simulink model "hexacopter_sim"  (R2024b)
settings: Solver=VariableStepAuto  StartTime=0  StopTime=100  FixedStep=0.1  RelTol=1e-3  EnableMultiTasking=on
values from neighbouring files (symbols this model uses):
  A = [zeros(4), eye(4); zeros(4),zeros(4)]    [hexacopter_par.m]
  b = 1.177*10^-5    (= 1.177e-05)    [hexacopter_par.m]
  B = [zeros(4) ... (first row only)    [hexacopter_par.m]
  C_obs = eye(8)    [hexacopter_par.m]
  d = 1.855*10^-7    (= 1.855e-07)    [hexacopter_par.m]
  fault_level = 0    [hexacopter_par.m]
  g = 9.81    [hexacopter_par.m]
  Ic = Ic + temp    [hexacopter_par.m]
  Ix = Ic(1,1)    [hexacopter_par.m]
  Iy = Ic(2,2)    [hexacopter_par.m]
  Iz = Ic(3,3)    [hexacopter_par.m]
  J_T = 1/2 *m_r* R_r^2    (= 0.0001)    [hexacopter_par.m]
  K_lqr = lqr(A', C_obs', Q, R)'    [hexacopter_par.m]
  K_phi = 0.03    [hexacopter_par.m]
  K_psi = 0.1    [hexacopter_par.m]
  K_theta = 0.03    [hexacopter_par.m]
  Kx = .1    (= 0.1)    [hexacopter_par.m]
  Ky = .1    (= 0.1)    [hexacopter_par.m]
  Kz = .1    (= 0.1)    [hexacopter_par.m]
  L = 0.275    [hexacopter_par.m]
  m = 2.5    [hexacopter_par.m]
  M_RB = [ m*eye(3) , zeros(3) ; zeros(3) , Ic ]    [hexacopter_par.m]
  motor_index = 3    [hexacopter_par.m]
  T_psinv = pinv(T)    [hexacopter_par.m]
libraries: slpidlib x19, simulink_extras x17, aerolibutil x2, matrix_library x2, vrlib x2, slctrl_smc x1
(part 3 of 3)

== system hexacopter_sim/Flight Control System1/Outer loop position control ==
  Pos. refs : Inport
  eta : Inport  Port=2
  Demux : Demux
  Demux1 : Demux  Outputs=6
  Demux2 : Demux  Outputs=2
  Gain : Gain  Gain=-1
  MATLAB Function : MATLAB Function  TreatAsAtomicUnit=on
  Mux : Mux
  Mux1 : Mux  Inputs=2
  PID Controller : slpidlib/PID Controller  Controller=PID  Form=Parallel  TimeDomain=Continuous-time  UseExternalTs=off  SampleTime=-1  IntegratorMethod=Forward Euler  FilterMethod=Forward Euler  ControllerParametersSource=internal  P=10  I=0  UseKiTs=off  D=35  UseExternalDerivativeSource=off  N=110  UseFilter=on  TunerSelectOption=Transfer Function Based (PID Tuner App)  InitialConditionSource=internal  InitialConditionForIntegrator=0  InitialConditionForFilter=0  DifferentiatorICPrevScaledInput=0  ExternalReset=none  TrackingMode=off  Kt=1  LimitOutput=off  SatLimitsSource=internal  UpperSaturationLimit=100  LowerSaturationLimit=-100  LinearizeAsGain=on  AntiWindupMode=none  Kb=1  LimitIntegrator=off  UpperIntegratorSaturationLimit=inf  LowerIntegratorSaturationLimit=-inf  POutMin=[]  POutMax=[]  IOutMin=[]  IOutMax=[]  DOutMin=[]  DOutMax=[]  NOutMin=[]  NOutMax=[]  SumOutMin=[]  SumOutMax=[]  SaturationOutMin=[]  SaturationOutMax=[]  PParamMin=[]  PParamMax=[]  IParamMin=[]  IParamMax=[]  DParamMin=[]  DParamMax=[]  NParamMin=[]  NParamMax=[]  KbParamMin=[]  KbParamMax=[]  KtParamMin=[]  KtParamMax=[]  KbOutMin=[]  KbOutMax=[]  KtOutMin=[]  KtOutMax=[]  IntegratorOutMin=[]  IntegratorOutMax=[]  FilterOutMin=[]  FilterOutMax=[]  SumI1OutMin=[]  SumI1OutMax=[]  SumI2OutMin=[]  SumI2OutMax=[]  SumI3OutMin=[]  SumI3OutMax=[]  SumI4OutMin=[]  SumI4OutMax=[]  SumDOutMin=[]  SumDOutMax=[]  DifferentiatorOutMin=[]  DifferentiatorOutMax=[]  FilterDiffOutCoefMin=[]  FilterDiffOutCoefMax=[]  ReciprocalOutMin=[]  ReciprocalOutMax=[]  SumDenOutMin=[]  SumDenOutMax=[]  SumNumOutMin=[]  SumNumOutMax=[]  DivideOutMin=[]  DivideOutMax=[]  UdiffTsProdOutMin=[]  UdiffTsProdOutMax=[]  NTsProdOutMin=[]  NTsProdOutMax=[]  UintegralTsProdOutMin=[]  UintegralTsProdOutMax=[]  UngainTsProdOutMin=[]  UngainTsProdOutMax=[]  ClampingZeroOutDataTypeStr=Inherit: Inherit via back propagation  ClampingZeroOutMin=[]  ClampingZeroOutMax=[]  FilterDenConstantOutDataTypeStr=Inherit: Inherit via back propagation  FilterDenConstantOutMin=[]  FilterDenConstantOutMax=[]  PCopyOutDataTypeStr=Inherit: Inherit via back propagation  PCopyOutMin=[]  PCopyOutMax=[]  NCopyOutDataTypeStr=Inherit: Inherit via back propagation  NCopyOutMin=[]  NCopyOutMax=[]  IntegratorContinuousStateAttributes=''  IntegratorStateMustResolveToSignalObject=off  IntegratorRTWStateStorageClass=Auto  FilterContinuousStateAttributes=''  FilterStateMustResolveToSignalObject=off  FilterRTWStateStorageClass=Auto  ParallelPVariant=InternalParameters  IdealPVariant=Disabled  IVariant=InternalParameters  DVariant=InternalParameters  IntegratorVariant=Continuous  SatVariant=Disabled  AWVariant=Passthrough  PCopyVariant=Disabled  TRVariant=Disabled  FdbkBlocksVariant=Forward  IdealPFdbkVariant=Disabled  SatFdbkVariant=Disabled  DerivativeFilterVariant=ContFilter  NVariant=InternalParameters  NCopyVariant=Disabled  FilterICVariant=InternalICsFilter  IntegratorICVariant=InternalICs  ExternalResetVariant=Disabled  TRSumVariant=Passthrough  SumFdbkVariant=Disabled  SumVariant=Sum_PID  TsampFilterVariant=InternalTs  TsampNgainVariant=Passthrough  TsampIntegralVariant=Disabled_SignalSpec  ExternalSaturationOutDataTypeStr=Inherit: Same as second input  DerivativeSourceVariant=ErrorSignal  PreIntVariant=InternalPreInt
  PID Controller2 : slpidlib/PID Controller  Controller=PID  Form=Parallel  TimeDomain=Continuous-time  UseExternalTs=off  SampleTime=-1  IntegratorMethod=Forward Euler  FilterMethod=Forward Euler  ControllerParametersSource=internal  P=0.00012475905697814  I=1.47736767470013e-06  UseKiTs=off  D=0.00234086595699177  UseExternalDerivativeSource=off  N=231.972359946857  UseFilter=on  TunerSelectOption=Transfer Function Based (PID Tuner App)  InitialConditionSource=internal  InitialConditionForIntegrator=0  InitialConditionForFilter=0  DifferentiatorICPrevScaledInput=0  ExternalReset=none  TrackingMode=off  Kt=1  LimitOutput=off  SatLimitsSource=internal  UpperSaturationLimit=100  LowerSaturationLimit=-100  LinearizeAsGain=on  AntiWindupMode=none  Kb=1  LimitIntegrator=off  UpperIntegratorSaturationLimit=inf  LowerIntegratorSaturationLimit=-inf  POutMin=[]  POutMax=[]  IOutMin=[]  IOutMax=[]  DOutMin=[]  DOutMax=[]  NOutMin=[]  NOutMax=[]  SumOutMin=[]  SumOutMax=[]  SaturationOutMin=[]  SaturationOutMax=[]  PParamMin=[]  PParamMax=[]  IParamMin=[]  IParamMax=[]  DParamMin=[]  DParamMax=[]  NParamMin=[]  NParamMax=[]  KbParamMin=[]  KbParamMax=[]  KtParamMin=[]  KtParamMax=[]  KbOutMin=[]  KbOutMax=[]  KtOutMin=[]  KtOutMax=[]  IntegratorOutMin=[]  IntegratorOutMax=[]  FilterOutMin=[]  FilterOutMax=[]  SumI1OutMin=[]  SumI1OutMax=[]  SumI2OutMin=[]  SumI2OutMax=[]  SumI3OutMin=[]  SumI3OutMax=[]  SumI4OutMin=[]  SumI4OutMax=[]  SumDOutMin=[]  SumDOutMax=[]  DifferentiatorOutMin=[]  DifferentiatorOutMax=[]  FilterDiffOutCoefMin=[]  FilterDiffOutCoefMax=[]  ReciprocalOutMin=[]  ReciprocalOutMax=[]  SumDenOutMin=[]  SumDenOutMax=[]  SumNumOutMin=[]  SumNumOutMax=[]  DivideOutMin=[]  DivideOutMax=[]  UdiffTsProdOutMin=[]  UdiffTsProdOutMax=[]  NTsProdOutMin=[]  NTsProdOutMax=[]  UintegralTsProdOutMin=[]  UintegralTsProdOutMax=[]  UngainTsProdOutMin=[]  UngainTsProdOutMax=[]  ClampingZeroOutDataTypeStr=Inherit: Inherit via back propagation  ClampingZeroOutMin=[]  ClampingZeroOutMax=[]  FilterDenConstantOutDataTypeStr=Inherit: Inherit via back propagation  FilterDenConstantOutMin=[]  FilterDenConstantOutMax=[]  PCopyOutDataTypeStr=Inherit: Inherit via back propagation  PCopyOutMin=[]  PCopyOutMax=[]  NCopyOutDataTypeStr=Inherit: Inherit via back propagation  NCopyOutMin=[]  NCopyOutMax=[]  IntegratorContinuousStateAttributes=''  IntegratorStateMustResolveToSignalObject=off  IntegratorRTWStateStorageClass=Auto  FilterContinuousStateAttributes=''  FilterStateMustResolveToSignalObject=off  FilterRTWStateStorageClass=Auto  ParallelPVariant=InternalParameters  IdealPVariant=Disabled  IVariant=InternalParameters  DVariant=InternalParameters  IntegratorVariant=Continuous  SatVariant=Disabled  AWVariant=Passthrough  PCopyVariant=Disabled  TRVariant=Disabled  FdbkBlocksVariant=Forward  IdealPFdbkVariant=Disabled  SatFdbkVariant=Disabled  DerivativeFilterVariant=ContFilter  NVariant=InternalParameters  NCopyVariant=Disabled  FilterICVariant=InternalICsFilter  IntegratorICVariant=InternalICs  ExternalResetVariant=Disabled  TRSumVariant=Passthrough  SumFdbkVariant=Disabled  SumVariant=Sum_PID  TsampFilterVariant=InternalTs  TsampNgainVariant=Passthrough  TsampIntegralVariant=Disabled_SignalSpec  ExternalSaturationOutDataTypeStr=Inherit: Same as second input  DerivativeSourceVariant=ErrorSignal  PreIntVariant=InternalPreInt
  Sum : Sum  Inputs=|+-
  Sum1 : Sum  Inputs=|+-
  Terminator : Terminator
  Terminator1 : Terminator
  Terminator2 : Terminator
  desired z,phi,theta,psi : Outport
  wires:
  Demux1/6 -> MATLAB Function/2(psi)
  Demux1/5 -> Terminator2/1
  Demux2/2 -> PID Controller2/1
  Demux2/1 -> PID Controller/1
  Mux1/1 -> MATLAB Function/1(Deltap_e)
  MATLAB Function/1(Deltap_b) -> Demux2/1
  Sum1/1 -> Mux1/2
  Sum/1 -> Mux1/1
  Demux/2 -> Sum1/1
  Demux/1 -> Sum/1
  Demux/4 -> Mux/4
  Demux/3 -> Mux/1
  PID Controller2/1 -> Mux/2
  Gain/1 -> Mux/3
  PID Controller/1 -> Gain/1
  Mux/1 -> desired z,phi,theta,psi/1
  eta/1 -> Demux1/1
  Demux1/1 -> Sum/2
  Demux1/4 -> Terminator1/1
  Demux1/2 -> Sum1/2
  Pos. refs/1 -> Demux/1
  Demux1/3 -> Terminator/1

== system hexacopter_sim/Formatting/Axes to VR Axes ==
  Xe : Inport
  Demux : Demux  Outputs=3
      settings: DisplayOption=none
  Mux : Mux  Inputs=3
  rad-->deg1 : Gain  SaturateOnIntegerOverflow=on  OutDataTypeStr=Inherit: Same as input  ParamDataTypeStr=Inherit: Same as input
  Xe VR : Outport  VectorParamsAs1DForOutWhenUnconnected=off
  wires:
  Xe/1 -> Demux/1
  Demux/1 -> Mux/1
  Demux/3 -> rad-->deg1/1
  Mux/1 -> Xe VR/1
  Demux/2 -> Mux/2
  rad-->deg1/1 -> Mux/3

== system hexacopter_sim/Formatting/Euler to VR ==
  Euler Angles : Inport
  Axis Angle Vector : Subsystem
  Mux : Mux  Inputs=2
  Mux1 : Mux  Inputs=2
  Mux2 : Mux  Inputs=2
  Quaternion Multiplication (Pitch & Yaw) : aerolibutil/Quaternion Multiplication
  Quaternion Multiplication (Roll) : aerolibutil/Quaternion Multiplication
  Quaternion Normalization : Subsystem
  Quaternion Normalization1 : Subsystem
  Quaternion Normalization2 : Subsystem
  Selector : Selector  InputPortWidth=3  IndexOptions=Index vector (dialog)  Indices=[3]  OutputSizes=1
  Selector1 : Selector  InputPortWidth=3  IndexOptions=Index vector (dialog)  Indices=[2]  OutputSizes=1
  Selector2 : Selector  InputPortWidth=3  IndexOptions=Index vector (dialog)  Indices=[1]  OutputSizes=1
  Vr Pitch Axes : Constant  Value=[0 0 1]
  Vr Roll Axes : Constant  Value=[1 0 0]
  Vr Yaw Axes : Constant  Value=[0 -1 0]
  Axis Angle : Outport  VectorParamsAs1DForOutWhenUnconnected=off
  wires:
  Quaternion Multiplication (Roll)/1 -> Axis Angle Vector/1(e0)
  Axis Angle Vector/1(e0_norm) -> Axis Angle/1
  Quaternion Normalization/1(e0_norm) -> Quaternion Multiplication (Roll)/2
  Quaternion Normalization2/1(e0_norm) -> Quaternion Multiplication (Pitch & Yaw)/1
  Quaternion Normalization1/1(e0_norm) -> Quaternion Multiplication (Pitch & Yaw)/2
  Mux2/1 -> Quaternion Normalization2/1(e0)
  Mux1/1 -> Quaternion Normalization1/1(e0)
  Mux/1 -> Quaternion Normalization/1(e0)
  Selector/1 -> Mux2/1
  Vr Yaw Axes/1 -> Mux2/2
  Selector1/1 -> Mux1/1
  Vr Pitch Axes/1 -> Mux1/2
  Selector2/1 -> Mux/1
  Vr Roll Axes/1 -> Mux/2
  Euler Angles/1 -> Selector2/1, Selector1/1, Selector/1
  Quaternion Multiplication (Pitch & Yaw)/1 -> Quaternion Multiplication (Roll)/1

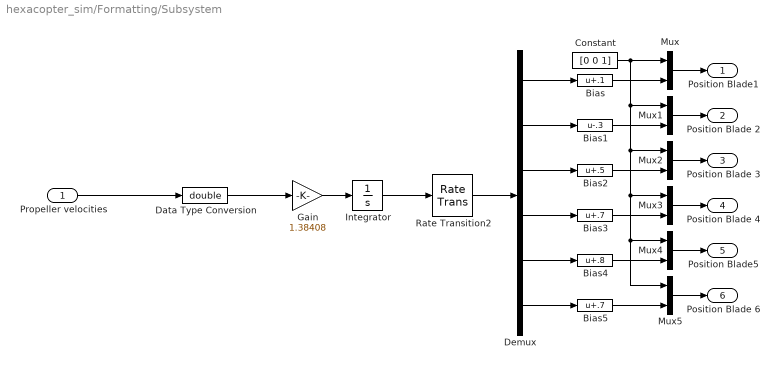
== system hexacopter_sim/Formatting/Subsystem ==
  Propeller velocities : Inport
  Bias : Bias  Bias=.1  SaturateOnIntegerOverflow=off
  Bias1 : Bias  Bias=-.3  SaturateOnIntegerOverflow=off
  Bias2 : Bias  Bias=.5  SaturateOnIntegerOverflow=off
  Bias3 : Bias  Bias=.7  SaturateOnIntegerOverflow=off
  Bias4 : Bias  Bias=.8  SaturateOnIntegerOverflow=off
  Bias5 : Bias  Bias=.7  SaturateOnIntegerOverflow=off
  Constant : Constant  Value=[0 0 1]
  Data Type Conversion : DataTypeConversion  OutDataTypeStr=double  SaturateOnIntegerOverflow=off  RndMeth=Floor
  Demux : Demux  Outputs=6
  Gain : Gain  Gain=1.38408
  Integrator : Integrator  InitialCondition=[.1 ; .2 ;-.3 ;-.4;.5;.6]  WrapState=on  WrappedStateUpperValue=2*pi  WrappedStateLowerValue=-2*pi
  Mux{,1..5} (6 alike) : Mux  Inputs=2
  Rate Transition2 : RateTransition
  Position Blade1 : Outport  VectorParamsAs1DForOutWhenUnconnected=off
  Position Blade 2 : Outport  Port=2  VectorParamsAs1DForOutWhenUnconnected=off
  Position Blade 3 : Outport  Port=3  VectorParamsAs1DForOutWhenUnconnected=off
  Position Blade 4 : Outport  Port=4  VectorParamsAs1DForOutWhenUnconnected=off
  Position Blade5 : Outport  Port=5  VectorParamsAs1DForOutWhenUnconnected=off
  Position Blade 6 : Outport  Port=6  VectorParamsAs1DForOutWhenUnconnected=off
  wires:
  Bias3/1 -> Mux3/2
  Mux3/1 -> Position Blade 4/1
  Bias1/1 -> Mux1/2
  Bias2/1 -> Mux2/2
  Demux/2 -> Bias1/1
  Constant/1 -> Mux4/1, Mux5/1, Mux3/1, Mux2/1, Mux1/1, Mux/1
  Mux1/1 -> Position Blade 2/1
  Mux2/1 -> Position Blade 3/1
  Integrator/1 -> Rate Transition2/1
  Mux/1 -> Position Blade1/1
  Demux/3 -> Bias2/1
  Bias/1 -> Mux/2
  Propeller velocities/1 -> Data Type Conversion/1
  Demux/4 -> Bias3/1
  Rate Transition2/1 -> Demux/1
  Demux/1 -> Bias/1
  Data Type Conversion/1 -> Gain/1
  Gain/1 -> Integrator/1
  Mux4/1 -> Position Blade5/1
  Mux5/1 -> Position Blade 6/1
  Demux/5 -> Bias4/1
  Demux/6 -> Bias5/1
  Bias5/1 -> Mux5/2
  Bias4/1 -> Mux4/2

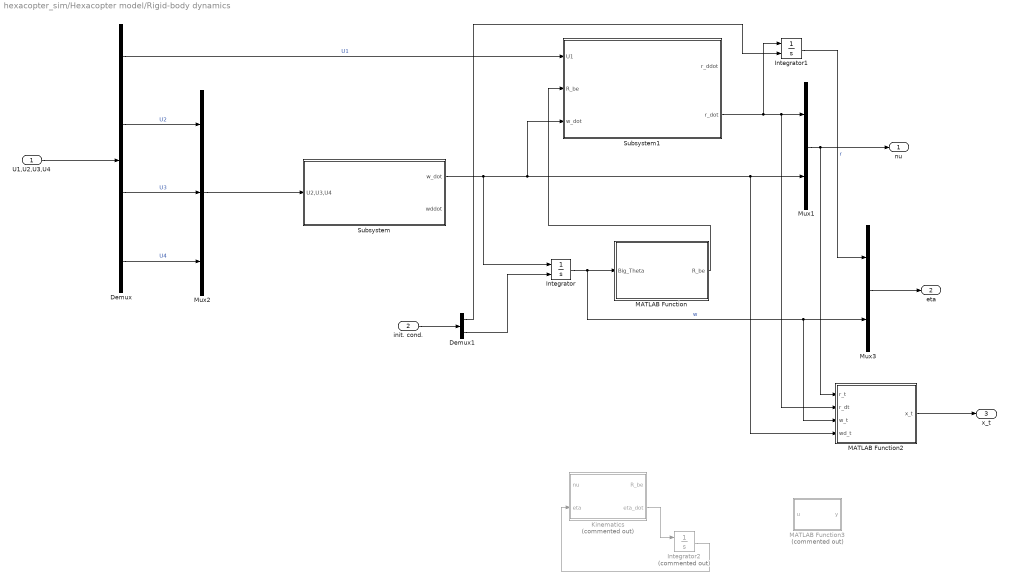
== system hexacopter_sim/Hexacopter model/Rigid-body dynamics ==
  U1,U2,U3,U4 : Inport
  init. cond. : Inport  Port=2
  Demux : Demux
  Demux1 : Demux  Outputs=2
  Integrator : Integrator  InitialConditionSource=external
  Integrator1 : Integrator  InitialConditionSource=external
  Integrator2 : Integrator  Commented=on  InitialConditionSource=external  InitialCondition=[0;0;-10;0;pi/2;0]
  Kinematics : MATLAB Function  Commented=on  TreatAsAtomicUnit=on
  MATLAB Function : MATLAB Function  TreatAsAtomicUnit=on
  MATLAB Function2 : MATLAB Function  TreatAsAtomicUnit=on
  MATLAB Function3 : MATLAB Function  Commented=on  TreatAsAtomicUnit=on
  Mux1 : Mux  Inputs=2
  Mux2 : Mux  Inputs=3
  Mux3 : Mux  Inputs=2
  Subsystem : Subsystem
  Subsystem1 : Subsystem
  nu : Outport
  eta : Outport  Port=2
  x_t : Outport  Port=3
  wires:
  U1,U2,U3,U4/1 -> Demux/1
  Demux/2 -> Mux2/1  "U2"
  Demux/3 -> Mux2/2  "U3"
  Demux/4 -> Mux2/3  "U4"
  Mux1/1 -> MATLAB Function2/1(r_t), nu/1
  Mux2/1 -> Subsystem/1(U2,U3,U4)
  Demux/1 -> Subsystem1/1(U1)  "U1"
  Subsystem/1(w_dot) -> Integrator/1, Subsystem1/3(w_dot), MATLAB Function2/4(wd_t), Mux1/2
  Subsystem1/2(r_dot) -> Integrator1/1, MATLAB Function2/2(r_dt), Mux1/1
  Integrator/1 -> MATLAB Function2/3(w_t), Mux3/2, MATLAB Function/1(Big_Theta)  "w"
  MATLAB Function/1(R_be) -> Subsystem1/2(R_be)
  Integrator1/1 -> Mux3/1  "r"
  Mux3/1 -> eta/1
  init. cond./1 -> Demux1/1
  Demux1/2 -> Integrator/2
  Demux1/1 -> Integrator1/2
  MATLAB Function2/1(x_t) -> x_t/1
  Integrator2/1 -> Kinematics/2(eta)
  Kinematics/2(eta_dot) -> Integrator2/1

== system hexacopter_sim/Observer - Allocation Matrix/U1 ==
  Fi : Inport
  Demux : Demux  Outputs=6
  Sum of Elements : Sum  Inputs=++++++
  U1 : Outport
  wires:
  Fi/1 -> Demux/1
  Demux/2 -> Sum of Elements/2  "F2"
  Demux/1 -> Sum of Elements/1  "F1"
  Demux/3 -> Sum of Elements/3  "F3"
  Demux/4 -> Sum of Elements/4  "F4"
  Demux/5 -> Sum of Elements/5  "F5"
  Demux/6 -> Sum of Elements/6  "F6"
  Sum of Elements/1 -> U1/1

== system hexacopter_sim/Observer - Allocation Matrix/U2 ==
  Fi : Inport
  Demux : Demux  Outputs=6
  Gain : Gain  Gain=1/2
  Gain1 : Gain  Gain=L
  Sum : Sum  Inputs=|-+
  Sum of Elements : Sum  Inputs=-++-
  Sum1 : Sum  Inputs=|++
  U2 : Outport
  wires:
  Fi/1 -> Demux/1
  Demux/1 -> Sum/1  "F1"
  Demux/6 -> Sum of Elements/4  "F6"
  Demux/5 -> Sum of Elements/3  "F5"
  Sum of Elements/1 -> Gain/1
  Sum/1 -> Sum1/1
  Gain/1 -> Sum1/2
  Sum1/1 -> Gain1/1
  Gain1/1 -> U2/1
  Demux/2 -> Sum of Elements/1  "F2"
  Demux/4 -> Sum/2  "F4"
  Demux/3 -> Sum of Elements/2  "F3"

== system hexacopter_sim/Observer - Allocation Matrix/U3 ==
  Fi : Inport
  Demux : Demux  Outputs=6
  Gain : Gain  Gain=L/2*sqrt(3)
  Sum of Elements : Sum  Inputs=++--
  Terminator : Terminator
  Terminator1 : Terminator
  U3 : Outport
  wires:
  Sum of Elements/1 -> Gain/1
  Demux/5 -> Sum of Elements/3  "F5"
  Demux/6 -> Sum of Elements/4  "F6"
  Fi/1 -> Demux/1
  Demux/1 -> Terminator/1  "F1"
  Demux/2 -> Sum of Elements/1  "F2"
  Gain/1 -> U3/1
  Demux/4 -> Terminator1/1  "F4"
  Demux/3 -> Sum of Elements/2  "F3"

== system hexacopter_sim/Observer - Allocation Matrix/U4 ==
  Tau_i : Inport
  Demux : Demux  Outputs=6
  Sum of Elements : Sum  Inputs=-+--++
  U4 : Outport
  wires:
  Tau_i/1 -> Demux/1
  Sum of Elements/1 -> U4/1
  Demux/1 -> Sum of Elements/1  "Tau_1"
  Demux/2 -> Sum of Elements/2  "Tau_2"
  Demux/3 -> Sum of Elements/3  "Tau_3"
  Demux/4 -> Sum of Elements/4  "Tau_4"
  Demux/5 -> Sum of Elements/5  "Tau_5"
  Demux/6 -> Sum of Elements/6  "Tau_6"

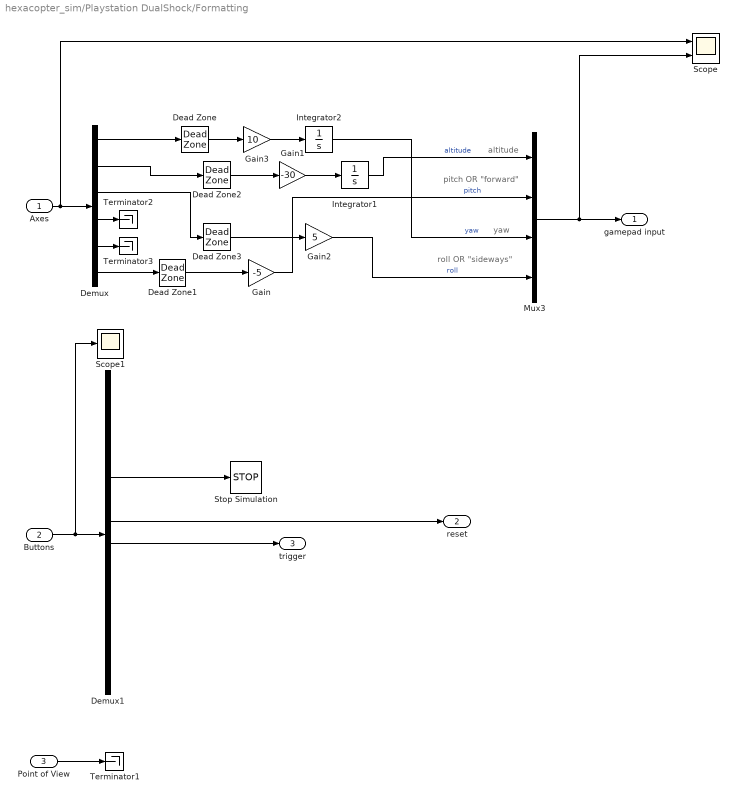
== system hexacopter_sim/Playstation DualShock/Formatting ==
  note: roll OR "sideways"
  note: altitude
  note: pitch OR "forward"
  note: yaw
  Axes : Inport
  Buttons : Inport  Port=2
  Point of View : Inport  Port=3
  Dead Zone{,1..3} (4 alike) : DeadZone  LowerValue=-0.2  UpperValue=0.2
  Demux : Demux  Outputs=6
  Demux1 : Demux  Outputs=14
  Gain : Gain  Gain=-5
  Gain1 : Gain  Gain=-30
  Gain2 : Gain  Gain=5
  Gain3 : Gain  Gain=10
  Integrator1 : Integrator  InitialCondition=10
  Integrator2 : Integrator
  Mux3 : Mux
  Scope : Scope  NumInputPorts=2
  Scope1 : Scope
  Stop Simulation : Stop
  Terminator1 : Terminator
  Terminator2 : Terminator
  Terminator3 : Terminator
  gamepad input : Outport
  reset : Outport  Port=2
  trigger : Outport  Port=3
  wires:
  Mux3/1 -> Scope/2, gamepad input/1
  Axes/1 -> Scope/1, Demux/1
  Demux/1 -> Dead Zone/1
  Dead Zone1/1 -> Gain/1
  Demux/2 -> Dead Zone2/1
  Dead Zone2/1 -> Gain1/1
  Dead Zone/1 -> Gain3/1
  Dead Zone3/1 -> Gain2/1
  Point of View/1 -> Terminator1/1
  Gain1/1 -> Integrator1/1
  Gain3/1 -> Integrator2/1
  Demux/3 -> Dead Zone3/1
  Integrator1/1 -> Mux3/1  "altitude"
  Gain2/1 -> Mux3/4  "roll"
  Gain/1 -> Mux3/2  "pitch"
  Integrator2/1 -> Mux3/3  "yaw"
  Demux/6 -> Dead Zone1/1
  Demux/4 -> Terminator2/1
  Demux/5 -> Terminator3/1
  Buttons/1 -> Scope1/1, Demux1/1
  Demux1/8 -> trigger/1
  Demux1/7 -> reset/1
  Demux1/5 -> Stop Simulation/1

== system hexacopter_sim/Quadcopter model/Kinematics ==
  nu : Inport
  init. cond. : Inport  Port=2
  Integrator : Integrator  InitialConditionSource=external  InitialCondition=[0;0;-10;0;pi/2;0]
  Kinematics : MATLAB Function  TreatAsAtomicUnit=on
  R_be : Outport
  eta : Outport  Port=2
  wires:
  Kinematics/1(R_be) -> R_be/1
  Kinematics/2(eta_dot) -> Integrator/1
  nu/1 -> Kinematics/1(nu)
  init. cond./1 -> Integrator/2
  Integrator/1 -> eta/1, Kinematics/2(eta)

== system hexacopter_sim/Quadcopter model/Rigid-body dynamics ==
  note: $\nu$
  tau_g : Inport
  tau_p : Inport  Port=2
  Constant : Constant  Value=m
  Constant1 : Constant  Value=Ic  VectorParams1D=off
  Coriolis term : MATLAB Function  TreatAsAtomicUnit=on
  Gain : Gain  Gain=inv(M_RB)  Multiplication=Matrix(K*u) (u vector)
  Integrator1 : Integrator  InitialCondition=[0;0;0;0;0;0]
  Sum : Sum  Inputs=++-
  nu : Outport
  wires:
  Integrator1/1 -> nu/1, Coriolis term/1(nu)
  Constant/1 -> Coriolis term/2(m)
  Sum/1 -> Gain/1
  tau_p/1 -> Sum/2
  Coriolis term/1(Cnunu) -> Sum/3
  Constant1/1 -> Coriolis term/3(Ic)
  Gain/1 -> Integrator1/1
  tau_g/1 -> Sum/1

== system hexacopter_sim/Quadcopter model/gravity ==
  R_be : Inport
  Manual Switch : ManualSwitch
  Math Function : Math  Operator=transpose
  Matrix Multiply : Product  Multiplication=Matrix(*)
  Mux2 : Mux  Inputs=2
  gravity vector : Constant  Value=[0;0;-m*g]  VectorParams1D=off
  zeros : Constant  Value=[0;0;0]  VectorParams1D=off
  tau_g : Outport
  wires:
  Matrix Multiply/1 -> Manual Switch/1
  Manual Switch/1 -> Mux2/1
  Mux2/1 -> tau_g/1
  gravity vector/1 -> Matrix Multiply/2
  zeros/1 -> Mux2/2, Manual Switch/2
  Math Function/1 -> Matrix Multiply/1
  R_be/1 -> Math Function/1

== system hexacopter_sim/Formatting/Euler to VR/Axis Angle Vector ==
  e0 : Inport
  2 : Gain  Gain=2  SaturateOnIntegerOverflow=on  OutDataTypeStr=Inherit: Same as input  ParamDataTypeStr=Inherit: Same as input
  Constant : Constant  Value=1e-6
  Demux : Demux  Outputs=[1 3 ]
      settings: DisplayOption=none
  Mux : Mux  Inputs=2
  Product : Product  Inputs=*/  InputSameDT=on  SaturateOnIntegerOverflow=on  OutDataTypeStr=Inherit: Same as first input
  Switch : Switch  Criteria=u2 ~= 0  SaturateOnIntegerOverflow=off  InputSameDT=off
  Trigonometric Function : Trigonometry
  Trigonometric Function2 : Trigonometry  Operator=acos
  e0_norm : Outport  VectorParamsAs1DForOutWhenUnconnected=off
  wires:
  Demux/1 -> Trigonometric Function2/1
  Demux/2 -> Product/1
  Mux/1 -> e0_norm/1
  Product/1 -> Mux/1
  2/1 -> Mux/2
  Trigonometric Function/1 -> Switch/1, Switch/2
  Trigonometric Function2/1 -> Trigonometric Function/1, 2/1
  e0/1 -> Demux/1
  Constant/1 -> Switch/3
  Switch/1 -> Product/2

== system hexacopter_sim/Formatting/Euler to VR/Quaternion Normalization ==
  e0 : Inport
  1/2 : Gain  Gain=1/2  SaturateOnIntegerOverflow=on  OutDataTypeStr=Inherit: Same as input  ParamDataTypeStr=Inherit: Same as input
  Demux : Demux  Outputs=[1 3]
      settings: DisplayOption=none
  Mux : Mux  Inputs=2
  Product : Product  InputSameDT=on  SaturateOnIntegerOverflow=on  OutDataTypeStr=Inherit: Same as first input
  Trigonometric Function : Trigonometry
  Trigonometric Function1 : Trigonometry  Operator=cos
  e0_norm : Outport  VectorParamsAs1DForOutWhenUnconnected=off
  wires:
  Trigonometric Function1/1 -> Mux/1
  Demux/2 -> Product/2
  Demux/1 -> 1/2/1
  Mux/1 -> e0_norm/1
  Product/1 -> Mux/2
  Trigonometric Function/1 -> Product/1
  1/2/1 -> Trigonometric Function1/1, Trigonometric Function/1
  e0/1 -> Demux/1

== system hexacopter_sim/Formatting/Euler to VR/Quaternion Normalization1 ==
  e0 : Inport
  1/2 : Gain  Gain=1/2  SaturateOnIntegerOverflow=on  OutDataTypeStr=Inherit: Same as input  ParamDataTypeStr=Inherit: Same as input
  Demux : Demux  Outputs=[1 3]
      settings: DisplayOption=none
  Mux : Mux  Inputs=2
  Product : Product  InputSameDT=on  SaturateOnIntegerOverflow=on  OutDataTypeStr=Inherit: Same as first input
  Trigonometric Function : Trigonometry
  Trigonometric Function1 : Trigonometry  Operator=cos
  e0_norm : Outport  VectorParamsAs1DForOutWhenUnconnected=off
  wires:
  e0/1 -> Demux/1
  1/2/1 -> Trigonometric Function/1, Trigonometric Function1/1
  Trigonometric Function/1 -> Product/1
  Product/1 -> Mux/2
  Mux/1 -> e0_norm/1
  Demux/1 -> 1/2/1
  Demux/2 -> Product/2
  Trigonometric Function1/1 -> Mux/1

== system hexacopter_sim/Formatting/Euler to VR/Quaternion Normalization2 ==
  e0 : Inport
  1/2 : Gain  Gain=1/2  SaturateOnIntegerOverflow=on  OutDataTypeStr=Inherit: Same as input  ParamDataTypeStr=Inherit: Same as input
  Demux : Demux  Outputs=[1 3]
      settings: DisplayOption=none
  Mux : Mux  Inputs=2
  Product : Product  InputSameDT=on  SaturateOnIntegerOverflow=on  OutDataTypeStr=Inherit: Same as first input
  Trigonometric Function : Trigonometry
  Trigonometric Function1 : Trigonometry  Operator=cos
  e0_norm : Outport  VectorParamsAs1DForOutWhenUnconnected=off
  wires:
  Trigonometric Function1/1 -> Mux/1
  Demux/2 -> Product/2
  Demux/1 -> 1/2/1
  Mux/1 -> e0_norm/1
  Product/1 -> Mux/2
  Trigonometric Function/1 -> Product/1
  1/2/1 -> Trigonometric Function1/1, Trigonometric Function/1
  e0/1 -> Demux/1

== system hexacopter_sim/Hexacopter model/Rigid-body dynamics/Subsystem ==
  U2,U3,U4 : Inport
  Constant : Constant  Value=Ic
  Cross Product : matrix_library/Cross Product
  Integrator : Integrator  InitialCondition=[0;0;0]
  Matrix Multiply1 : Product  Multiplication=Matrix(*)
  Sum : Sum  Inputs=|+-
  w_dot : Outport
  wddot : Outport  Port=2
  wires:
  Sum/1 -> Matrix Multiply1/2, wddot/1, Integrator/1  "wddot"
  Cross Product/1 -> Sum/2
  Integrator/1 -> Cross Product/1, w_dot/1  "w_dot"
  U2,U3,U4/1 -> Sum/1
  Matrix Multiply1/1 -> Cross Product/2
  Constant/1 -> Matrix Multiply1/1

== system hexacopter_sim/Hexacopter model/Rigid-body dynamics/Subsystem1 ==
  U1 : Inport
  R_be : Inport  Port=2
  w_dot : Inport  Port=3
  Constant2 : Constant  Value=[0;0]  VectorParams1D=off
  Cross Product1 : matrix_library/Cross Product
  Gain : Gain  Gain=1/m
  Integrator : Integrator  InitialCondition=[0;0;0]
  Matrix Multiply : Product  Multiplication=Matrix(*)
  Mux : Mux  Inputs=2
  Sum of Elements : Sum  Inputs=+--
  gravity vector : Constant  Value=[0;0;m*g]  VectorParams1D=off
  r_ddot : Outport
  r_dot : Outport  Port=2
  wires:
  Sum of Elements/1 -> Cross Product1/1, Gain/1
  gravity vector/1 -> Sum of Elements/2
  Constant2/1 -> Mux/1
  Gain/1 -> Integrator/1, r_ddot/1  "r_ddot"
  Matrix Multiply/1 -> Sum of Elements/1
  Cross Product1/1 -> Sum of Elements/3
  U1/1 -> Mux/2
  w_dot/1 -> Cross Product1/2
  Integrator/1 -> r_dot/1
  Mux/1 -> Matrix Multiply/2
  R_be/1 -> Matrix Multiply/1  "R_be"

== matlab function hexacopter_sim/Hexacopter model/Rigid-body dynamics/MATLAB Function2 ==
  data: r_t input; r_dt input; w_t input; wd_t input; x_t output
function x_t = fcn(r_t,r_dt,w_t,wd_t)

% Extract position components
% x = r_t(1); % x-coordinate
% y = r_t(2); % y-coordinate
z = r_t(3); % z-coordinate

% Extract velocity components
% dx = r_dt(1); % x-velocity
% dy = r_dt(2); % y-velocity
dz = r_dt(3); % z-velocity

% Extract Euler angles (orientation)
phi   = w_t(1); % Roll angle
theta = w_t(2); % Pitch angle
psi   = w_t(3); % Yaw angle

% Extract angular velocities
dphi   = wd_t(1); % Roll rate
dtheta = wd_t(2); % Pitch rate
dpsi   = wd_t(3); % Yaw rate

x_t = [phi, dphi, theta, dtheta, psi, dpsi, z, dz]';

== matlab function hexacopter_sim/fault detection/MATLAB Function1 ==
  data: x_meas input; r output; x_hat input
function r = compute_residuals(x_meas, x_hat)
%COMPUTE_RESIDUALS Computes reordered residuals according to:
% r1 = φ - ϕ̂
% r2 = θ - θ̂
% r3 = ψ - ψ̂
% r4 = z - ẑ
% r5 = φ̇ - ϕ̇̂
% r6 = θ̇ - θ̇̂
% r7 = ψ̇ - ψ̇̂
% r8 = ż - ż̂

%   x_meas : 8x1 vector of measured states [phi, dphi, theta, dtheta, psi, dpsi, z, dz]
%   x_hat  : 8x1 vector of estimated states [phi_hat, dphi_hat, theta_hat, ...]


if length(x_meas) ~= 8 || length(x_hat) ~= 8
    error('Both x_meas and x_hat must be 8x1 vectors.');
end

% Index map based on your definition
r = [ ...
    x_meas(1) - x_hat(1);  % φ - φ̂
    x_meas(3) - x_hat(3);  % θ - θ̂
    x_meas(5) - x_hat(5);  % ψ - ψ̂
    x_meas(7) - x_hat(7);  % z - ẑ
    x_meas(2) - x_hat(2);  % φ̇ - φ̇̂
    x_meas(4) - x_hat(4);  % θ̇ - θ̇̂
    x_meas(6) - x_hat(6);  % ψ̇ - ψ̇̂
    x_meas(8) - x_hat(8);  % ż - ż̂
];

== matlab function hexacopter_sim/fault detection/MATLAB Function ==
  data: motor_fault output; controllable output; r input; faulty output; s output
function [motor_fault, controllable, faulty,s] = detect_motor_fault_block(r)
%DETECT_MOTOR_FAULT_BLOCK Detects motor faults based on residual thresholds.

% Defaults
motor_fault = int8(0);
controllable = true;
faulty = false;

% Fault isolation using residuals r5 to r8
tolerance = 0.1; % Define a small threshold
r(abs(r) < tolerance) = 0; % Set small values to zero
s = r(5:8); % Apply sign function

% Thresholds
H_i = [50; 50; 50; 70; 0.15; 0.35; 0.15; 0.15];
M_i = [100; 100; 300; 10; 0.15; 0.35; 0.15; .15] * -1;

% If any residual is outside bounds, declare fault
for i = 5:8
    if r(i) >= H_i(i) || r(i) <= M_i(i)
        faulty = true;
        % break;
    end
end

if faulty
    % Check for motor fault
    
    % Match fault pattern using if-else for clarity
    if    s(1) == -1  && s(2) == -1 && s(3) == -1 && s(4) == -1 
        motor_fault = int8(2);  % Motor 2 failure
    elseif s(1) == -1 && abs(s(2)) < 0.1 && s(3) == -1 && s(4) == -1
        motor_fault = int8(5);  % Motor 2 failure
    elseif s(1) == 1 && s(2) == 1 && s(3) == -1 && s(4) == -1
        motor_fault = int8(6);  % Motor 6 failure
    elseif s(1) == 1 && abs(s(2)) < 0.1 && s(3) == 1 && s(4) == -1
        motor_fault = int8(3);  % Motor 4 failure
    elseif s(1) < -5 && s(2) > 1 && s(3) > 1 && s(4) < -0.4
        motor_fault = int8(5);  % Motor 1 failure
    elseif s(1) == 0 && s(2) > 0.275 && s(3) < -0.275 && s(4) < -0.02
        motor_fault = int8(5);  % Motor 6 failure
    end

end


% Controllability: motors 1 and 6 make system uncontrollable
if motor_fault == 1 || motor_fault == 6
    controllable = false;
end
end

== matlab function hexacopter_sim/Hexacopter model/Rigid-body dynamics/MATLAB Function3 ==
  data: u input; y output
function y = fcn(u)

% Rotation matrix from body to inertial frame
R_xphi = [ 1 0 0 ; 0 cos(phi) -sin(phi) ; 0 sin(phi) cos(phi) ];
R_ytheta = [ cos(theta) 0 sin(theta) ; 0 1 0 ; -sin(theta) 0 cos(theta) ];
R_zpsi = [ cos(psi) -sin(psi) 0 ; sin(psi) cos(psi) 0 ; 0 0 1 ];

% rotation matrix
R_be = R_zpsi * R_ytheta * R_xphi;


% cphi = cos(phi);
% sphi = sin(phi);
% ctheta = cos(theta);
% stheta = sin(theta);
% cpsi = cos(psi);
% spsi = sin(psi);

y = u;

== matlab function hexacopter_sim/Flight Control System without Allocation Matrix/Outer loop position control/MATLAB Function ==
  data: Deltap_e input; Deltap_b output; psi input
function Deltap_b = fcn(Deltap_e,psi)

R = [ cos(psi) , -sin(psi) ;
      sin(psi) ,  cos(psi) ];

Deltap_b = R'*Deltap_e;

== matlab function hexacopter_sim/Flight Control System/Outer loop position control/MATLAB Function ==
  data: Deltap_e input; Deltap_b output; psi input
function Deltap_b = fcn(Deltap_e,psi)

R = [ cos(psi) , -sin(psi) ;
      sin(psi) ,  cos(psi) ];

Deltap_b = R'*Deltap_e;

== matlab function hexacopter_sim/Allocation Matrix/MATLAB Function1 ==
  data: trigger input; motor_index input; omega_sq input; fault_level input; omega_out output; reset input
function omega_out = inject_fault_gamepad(trigger, motor_index, omega_sq, fault_level, reset )

persistent fault_active

% Initialize persistent variable on first run
if isempty(fault_active)
    fault_active = false;
end

% Handle reset first
if reset == 1
    fault_active = false;

% Otherwise set fault if trigger is active
elseif trigger == 1
    fault_active = true;
end

% Apply fault if active
omega_out = omega_sq;
if fault_active && motor_index >= 1 && motor_index <= 6 && fault_level >= 0 && fault_level <= 1
    omega_out(motor_index) = fault_level * omega_sq(motor_index);
end

% Clamp to ensure non-negative motor speeds
omega_out = max(omega_out, 0);

== matlab function hexacopter_sim/Observer - Allocation Matrix/MATLAB Function ==
  settings: updateMethod=DISCRETE
  data: tau_ref input; T_psinv input; omega_sq output
function omega_sq = fcn(tau_ref,  T_psinv)
% function omega_sq = fcn(tau_ref, , faulty_motor, fault_level)

%#codegen
% tau_ref        : 4x1 desired force vector
% L, d, b        : physical constants



% Compute reduced omega_sq for active motors
omega_active_sq = T_psinv * tau_ref;

% Build full 6x1 vector with zero values for faulty motors
omega_sq = zeros(6,1);
active_motors = 1:6;
omega_sq(active_motors) = omega_active_sq;

% Ensure non-negativity

omega_sq = max(omega_sq, 0);

== matlab function hexacopter_sim/Flight Control System1/Outer loop position control/MATLAB Function ==
  data: Deltap_e input; Deltap_b output; psi input
function Deltap_b = fcn(Deltap_e,psi)

R = [ cos(psi) , -sin(psi) ;
      sin(psi) ,  cos(psi) ];

Deltap_b = R'*Deltap_e;

== matlab function hexacopter_sim/Allocation Matrix/MATLAB Function2 ==
  settings: updateMethod=DISCRETE
  data: faulty_motors input; fault_flag input; fault_location output; reset_flag input
function fault_location = persistent_fault_fcn(faulty_motors, fault_flag, reset_flag)
% PERSISTENT_FAULT_FCN Converts motor indices into a persistent 6x1 fault vector.
% Faults remain latched until explicitly reset and if fault_flag is true.
%
% Inputs:
%   faulty_motors - vector of motor indices that have failed (e.g., [1 3])
%   fault_flag    - logical scalar indicating if faults should be latched
%   reset_flag    - optional logical flag to reset all faults (default: false)
% Output:
%   fault_location - 6x1 binary vector with latched faults (e.g., [1; 0; 1; 0; 0; 0])

persistent fault_history

% Initialize persistent fault storage on first call
if isempty(fault_history)
    fault_history = zeros(6, 1);  % Stored as binary double vector
end

% Reset logic
if nargin >= 3 && reset_flag
    fault_history = zeros(6, 1);
end

% Only latch faults if fault_flag is true
if fault_flag
    valid_faults = unique(faulty_motors(faulty_motors >= 1 & faulty_motors <= 6));
    fault_history(valid_faults) = 1;
end

% Return current latched fault vector
fault_location = fault_history;

== matlab function hexacopter_sim/fault detection/MATLAB Function2 ==
  settings: updateMethod=DISCRETE
  data: u input; y output
function y = hold_first_nonzero(u)
% This function holds the first non-zero int8 value it receives
persistent first_value

if isempty(first_value) && u ~= int8(0)
    first_value = int8(u); % Store the first non-zero value as int8
end

if isempty(first_value)
    y = int8(0); % Default output before a non-zero value is received
else
    y = first_value; % Hold the first non-zero value
end

== matlab function hexacopter_sim/Quadcopter model/Rigid-body dynamics/Coriolis term ==
  data: nu input; Cnunu output; m input; Ic input
function Cnunu = fcn(nu,m,Ic)

v = nu(1:3);  % linear velocities (expressed in the body frame)
omega = nu(4:6); % angular velocities (expressed in the body frame)


Cnunu = [ cross(omega,m*v) ; -cross(Ic*omega,omega) ];

== matlab function hexacopter_sim/Allocation Matrix/MATLAB Function ==
  settings: updateMethod=DISCRETE
  data: tau_ref input; parameters input; faulty_motors input; omega_sq output; reset input
function omega_sq = fcn(tau_ref, parameters, faulty_motors, reset)
% function omega_sq = fcn(tau_ref, T_psinv, faulty_motor, fault_level)

%#codegen
% tau_ref        : 4x1 desired wrench vector
% L, d, b        : physical constants
% faulty_motors  : vector of faulty motor indices (1-based)
% reset          : scalar flag (1 = reset/recompute allocation matrix)

L = parameters(1);
d = parameters(2);
b = parameters(3);


persistent T_full last_faulty_motors T_psinv_reduced active_motors

% Initialize full allocation matrix once
if isempty(T_full)
    T_full = [
        1,    1,     1,    1,     1,    1;
       -L, -L/2,   L/2,   L,     L/2,  -L/2;
        0,  L*sqrt(3)/2,  L*sqrt(3)/2,  0, -L*sqrt(3)/2, -L*sqrt(3)/2;
       -d/b, d/b, -d/b, -d/b, d/b, d/b
    ];
end
    % 
    % T_full = [
    %     1,   1,  1,   1,  1,  1;
    %    -L,   L,  L/2, -L/2, -L/2,  L/2;
    %     0,   0,  L*sqrt(3)/2, -L*sqrt(3)/2, L*sqrt(3)/2, -L*sqrt(3)/2;
    %    -d/b, d/b, -d/b, -d/b, d/b, d/b
    % ];

% Initialize all persistent variables
if isempty(T_psinv_reduced)
    T_psinv_reduced = pinv(T_full); % Safe fallback
end
if isempty(last_faulty_motors)
    last_faulty_motors = zeros(6,1);
end
if isempty(active_motors)
    active_motors = 1:6;
end


% Update T_psinv_reduced only if faulty motors changed or reset requested
if reset || ~isequal(faulty_motors, last_faulty_motors)
    all_motors = 1:6;
    active_motors = setdiff(all_motors, find(faulty_motors)); % find indices of faulty motors
    T_reduced = T_full(:, active_motors);
    T_psinv_reduced = pinv(T_reduced);
    last_faulty_motors = faulty_motors;
end

% Compute reduced omega_sq for active motors
omega_active_sq = T_psinv_reduced * tau_ref;

% Build full 6x1 vector with zero values for faulty motors
omega_sq = zeros(6,1);
omega_sq(active_motors) = omega_active_sq;

% Ensure non-negativity

omega_sq = max(omega_sq, 0);

== matlab function hexacopter_sim/Quadcopter model/Kinematics/Kinematics ==
  data: R_be output; nu input; eta input; eta_dot output
function [R_be,eta_dot] = J_Theta(nu,eta)

% Euler angle extraction
phi = eta(4);
theta = eta(5);
psi = eta(6);

R_xphi = [ 1 0 0 ; 0 cos(phi) -sin(phi) ; 0 sin(phi) cos(phi) ];
R_ytheta = [ cos(theta) 0 sin(theta) ; 0 1 0 ; -sin(theta) 0 cos(theta) ];
R_zpsi = [ cos(psi) -sin(psi) 0 ; sin(psi) cos(psi) 0 ; 0 0 1 ];

% rotation matrix
R_be = R_zpsi * R_ytheta * R_xphi;

% angular velocity transformation
T_Theta = [ 1 sin(phi)*tan(theta) cos(phi)*tan(theta) ; 0 cos(phi) -sin(phi) ; 0 sin(phi)/cos(theta) cos(phi)/cos(theta) ];

J_Theta = [ R_be , zeros(3) ; zeros(3) , T_Theta ];

eta_dot = J_Theta*nu;

== matlab function hexacopter_sim/Hexacopter model/Rigid-body dynamics/Kinematics ==
  data: R_be output; nu input; eta input; eta_dot output
function [R_be,eta_dot] = J_Theta(nu,eta)

% Euler angle extraction
phi = eta(4);
theta = eta(5);
psi = eta(6);

R_xphi = [ 1 0 0 ; 0 cos(phi) -sin(phi) ; 0 sin(phi) cos(phi) ];
R_ytheta = [ cos(theta) 0 sin(theta) ; 0 1 0 ; -sin(theta) 0 cos(theta) ];
R_zpsi = [ cos(psi) -sin(psi) 0 ; sin(psi) cos(psi) 0 ; 0 0 1 ];

% rotation matrix
R_be = R_zpsi * R_ytheta * R_xphi;

% angular velocity transformation
T_Theta = [ 1 sin(phi)*tan(theta) cos(phi)*tan(theta) ; 0 cos(phi) -sin(phi) ; 0 sin(phi)/cos(theta) cos(phi)/cos(theta) ];

J_Theta = [ R_be , zeros(3) ; zeros(3) , T_Theta ];

eta_dot = J_Theta*nu;

== matlab function hexacopter_sim/Hexacopter model/Linear Acceleration ==
  data: r_dot input; U input; r_ddot output; par input; w_t input
function r_ddot  = fcn(r_dot,U,par,w_t)

U1 = U(1);
Kx = par(1);
Ky = par(2);
Kz = par(3);
m = par(4);
g = par(5);

% Euler angle extraction
% phi = w_t(1);
% theta = w_t(3);
% psi = w_t(2);

% % Euler angle extraction YZX
% phi = w_t(1); % pitch 
% psi = w_t(2); % yaw
% theta = w_t(3); % roll

phi   = w_t(1); % roll
theta = w_t(3); % pitch
psi   = w_t(2); % yaw


% Linear velocities
xdot = r_dot(1);
ydot = r_dot(2);
zdot = r_dot(3);

% Rotation matrix elements (body to inertial)
% Assuming standard aerospace convention ZYX
R13 = sin(phi)*sin(psi) + cos(phi)*cos(psi)*sin(theta);
R23 = cos(phi)*sin(psi)*sin(theta) - cos(psi)*sin(phi);
R33 = cos(phi)*cos(theta);

% Assuming standard aerospace convention XYZ
 % R13 =           sin(theta);
 % R23 = -cos(theta)*sin(phi);
 % R33 =  cos(phi)*cos(theta);


% Assuming standard aerospace convention YZX
% R13 = cos(phi)*sin(theta) + cos(theta)*sin(phi)*sin(psi);
% R23 =                                 -cos(psi)*sin(phi);
% R33 = cos(phi)*cos(theta) - sin(phi)*sin(psi)*sin(theta);


% Translational accelerations
x_ddot = (-U1*R13 - Kx*xdot)/m;
y_ddot = (U1*R23 - Ky*ydot)/m;
z_ddot = -g + (U1*R33 - Kz*zdot)/m;

r_ddot = [x_ddot; y_ddot; z_ddot];

== matlab function hexacopter_sim/Hexacopter model/Angular Acceleration  ==
  data: U_out output; U input; par input; omega_in input; w_ddot output; w_dot input
function [U_out,w_ddot] = fcn(U,par, omega_in,w_dot)

U2 = U(2);
U3 = U(3);
U4 = U(4);

Ix = par(1);
Iy = par(2);
Iz = par(3);
Jr_single_rotor = par(4);

Kphi = par(5);
Ktheta = par(6);
Kpsi = par(7);

phi_dot = w_dot(1);
theta_dot = w_dot(2);
psi_dot = w_dot(3);


Jr = 6 * Jr_single_rotor;  % Jr is per rotor

% From paper (incorrect for hexacopter):
% Omega = omega_in(3) + omega_in(4) - omega_in(1) - omega_in(2);

% For hexacopter (6 rotors):
Omega = omega_in(1) + omega_in(3) + omega_in(4) ...
      - omega_in(2) - omega_in(5) - omega_in(6);


% Angular accelerations
phi_ddot = (U2 + (Iy - Iz) * theta_dot * psi_dot - ...
    Jr * Omega * theta_dot - Kphi * phi_dot) / Ix;

theta_ddot = (U3 + (Iz - Ix) * phi_dot * psi_dot + ...
    Jr * Omega * phi_dot - Ktheta * theta_dot) / Iy;

psi_ddot = (U4 + (Ix - Iy) * phi_dot * theta_dot - ...
    Kpsi * psi_dot) / Iz;

w_ddot = [phi_ddot; theta_ddot; psi_ddot]; % roll accel, pitch accel, yaw accel
U_out = U;

== matlab function hexacopter_sim/Hexacopter model/Rigid-body dynamics/MATLAB Function ==
  data: Big_Theta input; R_be output
function R_be = Rb2e(Big_Theta)

% Euler angle extraction
phi = Big_Theta(1);
theta = Big_Theta(2);
psi = Big_Theta(3);

% Rotation matrix from body to inertial frame
R_xphi = [ 1 0 0 ; 0 cos(phi) -sin(phi) ; 0 sin(phi) cos(phi) ];
R_ytheta = [ cos(theta) 0 sin(theta) ; 0 1 0 ; -sin(theta) 0 cos(theta) ];
R_zpsi = [ cos(psi) -sin(psi) 0 ; sin(psi) cos(psi) 0 ; 0 0 1 ];

% rotation matrix
R_be = R_zpsi * R_ytheta * R_xphi;

== matlab function hexacopter_sim/Thau Observer/MATLAB Function ==
  data: misc input; omega_in input; xhat input; hx output
function hx = h_function(misc,omega_in,xhat)

% States
phidot = xhat(2);
thetadot = xhat(4);
psidot = xhat(6);


% Inputs
% Correct for hexacopter (6 rotors):
Omega = omega_in(1) - omega_in(2) + omega_in(3) + ...
omega_in(4) - omega_in(5) - omega_in(6);

% Constants 
Ix = misc(1);  
Iy = misc(2);
Iz = misc(3);
JT = 6 * misc(4); % for six rotors
g = misc(5);

% Nonlinear dynamics
hx = zeros(8,1);  % initialize

hx(5) = (thetadot*psidot*(Iy - Iz) - JT*thetadot*Omega)/Ix;
hx(6) = (phidot*psidot*(Iz - Ix) - JT*phidot*Omega)/Iy;
hx(7) = phidot*thetadot*(Ix - Iy)/Iz;
hx(8) = -g;

== matlab function hexacopter_sim/Hexacopter model/MATLAB Function2 ==
  data: r_t input; r_dt input; w_t input; wd_t input; x_t output
function x_t = fcn(r_t,r_dt,w_t,wd_t)

% Extract position components
% x = r_t(1); % x-coordinate
% y = r_t(2); % y-coordinate
z = r_t(3); % z-coordinate

% Extract velocity components
% dx = r_dt(1); % x-velocity
% dy = r_dt(2); % y-velocity
dz = r_dt(3); % z-velocity

% Extract Euler angles (orientation)
phi   = w_t(1); % Roll angle
theta = w_t(2); % Pitch angle
psi   = w_t(3); % Yaw angle

% Extract angular velocities
dphi   = wd_t(1); % Roll rate
dtheta = wd_t(2); % Pitch rate
dpsi   = wd_t(3); % Yaw rate

x_t = [phi, dphi, theta, dtheta, psi, dpsi, z, dz]';
